simulink model "busCreators01curr"  (R2025b)
settings: Solver=VariableStepAuto  StartTime=0.0  StopTime=10.0  RelTol=1e-3
undefined symbols (not defined in the file or in its folder): Ts
settings Model: Creator=gdudgeon  LastModifiedBy=gdudgeon
settings RTWCC: GPUComputeCapability=3.5

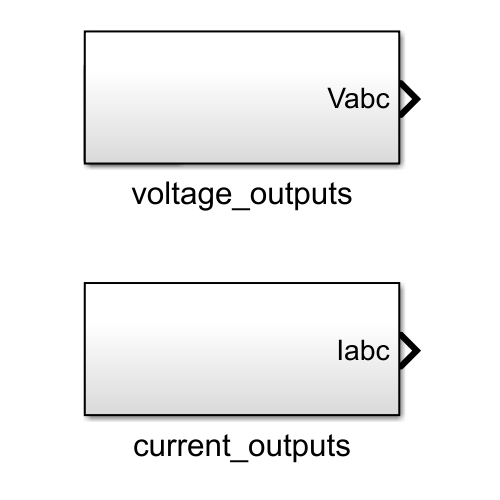
[thumbnail: Simulink's stored preview of the top-level diagram]
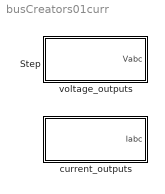
== system busCreators01curr ==
  Step : Step  SampleTime=0
  current_outputs : Subsystem
  voltage_outputs : Subsystem

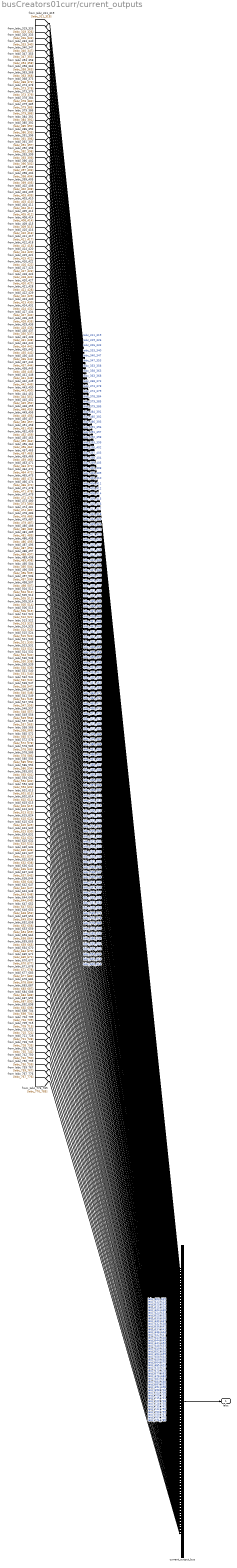
== system busCreators01curr/current_outputs ==
  current_output_bus : BusCreator  Inputs=169
  Iabc : Outport  SampleTime=Ts  VectorParamsAs1DForOutWhenUnconnected=off
  wires:
  [Iabc_776_785] -> current_output_bus/169  "Iabc_776_785"
  [Iabc_767_776] -> current_output_bus/168  "Iabc_767_776"
  [Iabc_759_767] -> current_output_bus/167  "Iabc_759_767"
  [Iabc_750_759] -> current_output_bus/166  "Iabc_750_759"
  [Iabc_742_750] -> current_output_bus/165  "Iabc_742_750"
  [Iabc_735_742] -> current_output_bus/164  "Iabc_735_742"
  [Iabc_728_735] -> current_output_bus/163  "Iabc_728_735"
  [Iabc_721_728] -> current_output_bus/162  "Iabc_721_728"
  [Iabc_715_721] -> current_output_bus/161  "Iabc_715_721"
  [Iabc_709_715] -> current_output_bus/160  "Iabc_709_715"
  [Iabc_704_709] -> current_output_bus/159  "Iabc_704_709"
  [Iabc_698_704] -> current_output_bus/158  "Iabc_698_704"
  [Iabc_692_698] -> current_output_bus/157  "Iabc_692_698"
  [Iabc_687_692] -> current_output_bus/156  "Iabc_687_692"
  [Iabc_684_688] -> current_output_bus/155  "Iabc_684_688"
  [Iabc_683_687] -> current_output_bus/154  "Iabc_683_687"
  [Iabc_678_684] -> current_output_bus/153  "Iabc_678_684"
  [Iabc_677_683] -> current_output_bus/152  "Iabc_677_683"
  [Iabc_671_678] -> current_output_bus/151  "Iabc_671_678"
  [Iabc_670_677] -> current_output_bus/150  "Iabc_670_677"
  [Iabc_665_671] -> current_output_bus/149  "Iabc_665_671"
  [Iabc_664_670] -> current_output_bus/148  "Iabc_664_670"
  [Iabc_659_665] -> current_output_bus/147  "Iabc_659_665"
  [Iabc_658_664] -> current_output_bus/146  "Iabc_658_664"
  [Iabc_653_659] -> current_output_bus/145  "Iabc_653_659"
  [Iabc_652_658] -> current_output_bus/144  "Iabc_652_658"
  [Iabc_649_654] -> current_output_bus/143  "Iabc_649_654"
  [Iabc_648_653] -> current_output_bus/142  "Iabc_648_653"
  [Iabc_647_652] -> current_output_bus/141  "Iabc_647_652"
  [Iabc_644_649] -> current_output_bus/140  "Iabc_644_649"
  [Iabc_643_648] -> current_output_bus/139  "Iabc_643_648"
  [Iabc_642_647] -> current_output_bus/138  "Iabc_642_647"
  [Iabc_638_644] -> current_output_bus/137  "Iabc_638_644"
  [Iabc_637_643] -> current_output_bus/136  "Iabc_637_643"
  [Iabc_636_642] -> current_output_bus/135  "Iabc_636_642"
  [Iabc_632_638] -> current_output_bus/134  "Iabc_632_638"
  [Iabc_631_637] -> current_output_bus/133  "Iabc_631_637"
  [Iabc_630_636] -> current_output_bus/132  "Iabc_630_636"
  [Iabc_625_632] -> current_output_bus/131  "Iabc_625_632"
  [Iabc_624_631] -> current_output_bus/130  "Iabc_624_631"
  [Iabc_623_630] -> current_output_bus/129  "Iabc_623_630"
  [Iabc_615_625] -> current_output_bus/128  "Iabc_615_625"
  [Iabc_615_624] -> current_output_bus/127  "Iabc_615_624"
  [Iabc_613_623] -> current_output_bus/126  "Iabc_613_623"
  [Iabc_603_615] -> current_output_bus/125  "Iabc_603_615"
  [Iabc_602_614] -> current_output_bus/124  "Iabc_602_614"
  [Iabc_601_613] -> current_output_bus/123  "Iabc_601_613"
  [Iabc_594_603] -> current_output_bus/122  "Iabc_594_603"
  [Iabc_594_602] -> current_output_bus/121  "Iabc_594_602"
  [Iabc_593_601] -> current_output_bus/120  "Iabc_593_601"
  [Iabc_586_594] -> current_output_bus/119  "Iabc_586_594"
  [Iabc_585_593] -> current_output_bus/118  "Iabc_585_593"
  [Iabc_578_586] -> current_output_bus/117  "Iabc_578_586"
  [Iabc_578_585] -> current_output_bus/116  "Iabc_578_585"
  [Iabc_572_578] -> current_output_bus/115  "Iabc_572_578"
  [Iabc_565_572] -> current_output_bus/114  "Iabc_565_572"
  [Iabc_558_566] -> current_output_bus/113  "Iabc_558_566"
  [Iabc_557_565] -> current_output_bus/112  "Iabc_557_565"
  [Iabc_549_558] -> current_output_bus/111  "Iabc_549_558"
  [Iabc_548_557] -> current_output_bus/110  "Iabc_548_557"
  [Iabc_547_556] -> current_output_bus/109  "Iabc_547_556"
  [Iabc_541_549] -> current_output_bus/108  "Iabc_541_549"
  [Iabc_540_548] -> current_output_bus/107  "Iabc_540_548"
  [Iabc_538_547] -> current_output_bus/106  "Iabc_538_547"
  [Iabc_532_541] -> current_output_bus/105  "Iabc_532_541"
  [Iabc_531_540] -> current_output_bus/104  "Iabc_531_540"
  [Iabc_530_539] -> current_output_bus/103  "Iabc_530_539"
  [Iabc_530_538] -> current_output_bus/102  "Iabc_530_538"
  [Iabc_524_532] -> current_output_bus/101  "Iabc_524_532"
  [Iabc_523_531] -> current_output_bus/100  "Iabc_523_531"
  [Iabc_521_530] -> current_output_bus/99  "Iabc_521_530"
  [Iabc_515_524] -> current_output_bus/98  "Iabc_515_524"
  [Iabc_514_523] -> current_output_bus/97  "Iabc_514_523"
  [Iabc_513_522] -> current_output_bus/96  "Iabc_513_522"
  [Iabc_512_521] -> current_output_bus/95  "Iabc_512_521"
  [Iabc_506_515] -> current_output_bus/94  "Iabc_506_515"
  [Iabc_505_514] -> current_output_bus/93  "Iabc_505_514"
  [Iabc_505_513] -> current_output_bus/92  "Iabc_505_513"
  [Iabc_504_512] -> current_output_bus/91  "Iabc_504_512"
  [Iabc_498_507] -> current_output_bus/90  "Iabc_498_507"
  [Iabc_497_506] -> current_output_bus/89  "Iabc_497_506"
  [Iabc_496_505] -> current_output_bus/88  "Iabc_496_505"
  [Iabc_495_504] -> current_output_bus/87  "Iabc_495_504"
  [Iabc_489_498] -> current_output_bus/86  "Iabc_489_498"
  [Iabc_488_497] -> current_output_bus/85  "Iabc_488_497"
  [Iabc_487_496] -> current_output_bus/84  "Iabc_487_496"
  [Iabc_486_495] -> current_output_bus/83  "Iabc_486_495"
  [Iabc_481_489] -> current_output_bus/82  "Iabc_481_489"
  [Iabc_480_488] -> current_output_bus/81  "Iabc_480_488"
  [Iabc_479_487] -> current_output_bus/80  "Iabc_479_487"
  [Iabc_478_486] -> current_output_bus/79  "Iabc_478_486"
  [Iabc_474_481] -> current_output_bus/78  "Iabc_474_481"
  [Iabc_473_480] -> current_output_bus/77  "Iabc_473_480"
  [Iabc_472_479] -> current_output_bus/76  "Iabc_472_479"
  [Iabc_471_478] -> current_output_bus/75  "Iabc_471_478"
  [Iabc_466_474] -> current_output_bus/74  "Iabc_466_474"
  [Iabc_465_473] -> current_output_bus/73  "Iabc_465_473"
  [Iabc_464_472] -> current_output_bus/72  "Iabc_464_472"
  [Iabc_463_471] -> current_output_bus/71  "Iabc_463_471"
  [Iabc_459_466] -> current_output_bus/70  "Iabc_459_466"
  [Iabc_457_465] -> current_output_bus/69  "Iabc_457_465"
  [Iabc_456_464] -> current_output_bus/68  "Iabc_456_464"
  [Iabc_455_463] -> current_output_bus/67  "Iabc_455_463"
  [Iabc_452_459] -> current_output_bus/66  "Iabc_452_459"
  [Iabc_451_458] -> current_output_bus/65  "Iabc_451_458"
  [Iabc_450_457] -> current_output_bus/64  "Iabc_450_457"
  [Iabc_449_456] -> current_output_bus/63  "Iabc_449_456"
  [Iabc_448_455] -> current_output_bus/62  "Iabc_448_455"
  [Iabc_445_452] -> current_output_bus/61  "Iabc_445_452"
  [Iabc_444_451] -> current_output_bus/60  "Iabc_444_451"
  [Iabc_443_450] -> current_output_bus/59  "Iabc_443_450"
  [Iabc_442_449] -> current_output_bus/58  "Iabc_442_449"
  [Iabc_441_448] -> current_output_bus/57  "Iabc_441_448"
  [Iabc_438_445] -> current_output_bus/56  "Iabc_438_445"
  [Iabc_437_444] -> current_output_bus/55  "Iabc_437_444"
  [Iabc_436_443] -> current_output_bus/54  "Iabc_436_443"
  [Iabc_435_442] -> current_output_bus/53  "Iabc_435_442"
  [Iabc_434_441] -> current_output_bus/52  "Iabc_434_441"
  [Iabc_431_438] -> current_output_bus/51  "Iabc_431_438"
  [Iabc_430_437] -> current_output_bus/50  "Iabc_430_437"
  [Iabc_429_436] -> current_output_bus/49  "Iabc_429_436"
  [Iabc_428_435] -> current_output_bus/48  "Iabc_428_435"
  [Iabc_427_434] -> current_output_bus/47  "Iabc_427_434"
  [Iabc_424_431] -> current_output_bus/46  "Iabc_424_431"
  [Iabc_423_430] -> current_output_bus/45  "Iabc_423_430"
  [Iabc_422_429] -> current_output_bus/44  "Iabc_422_429"
  [Iabc_421_428] -> current_output_bus/43  "Iabc_421_428"
  [Iabc_420_427] -> current_output_bus/42  "Iabc_420_427"
  [Iabc_418_424] -> current_output_bus/41  "Iabc_418_424"
  [Iabc_417_423] -> current_output_bus/40  "Iabc_417_423"
  [Iabc_416_422] -> current_output_bus/39  "Iabc_416_422"
  [Iabc_415_421] -> current_output_bus/38  "Iabc_415_421"
  [Iabc_414_420] -> current_output_bus/37  "Iabc_414_420"
  [Iabc_412_418] -> current_output_bus/36  "Iabc_412_418"
  [Iabc_411_417] -> current_output_bus/35  "Iabc_411_417"
  [Iabc_410_416] -> current_output_bus/34  "Iabc_410_416"
  [Iabc_409_415] -> current_output_bus/33  "Iabc_409_415"
  [Iabc_408_414] -> current_output_bus/32  "Iabc_408_414"
  [Iabc_405_412] -> current_output_bus/31  "Iabc_405_412"
  [Iabc_404_411] -> current_output_bus/30  "Iabc_404_411"
  [Iabc_403_410] -> current_output_bus/29  "Iabc_403_410"
  [Iabc_403_409] -> current_output_bus/28  "Iabc_403_409"
  [Iabc_402_408] -> current_output_bus/27  "Iabc_402_408"
  [Iabc_399_405] -> current_output_bus/26  "Iabc_399_405"
  [Iabc_398_404] -> current_output_bus/25  "Iabc_398_404"
  [Iabc_397_403] -> current_output_bus/24  "Iabc_397_403"
  [Iabc_396_402] -> current_output_bus/23  "Iabc_396_402"
  [Iabc_393_399] -> current_output_bus/22  "Iabc_393_399"
  [Iabc_392_398] -> current_output_bus/21  "Iabc_392_398"
  [Iabc_391_397] -> current_output_bus/20  "Iabc_391_397"
  [Iabc_391_396] -> current_output_bus/19  "Iabc_391_396"
  [Iabc_386_393] -> current_output_bus/18  "Iabc_386_393"
  [Iabc_385_392] -> current_output_bus/17  "Iabc_385_392"
  [Iabc_384_391] -> current_output_bus/16  "Iabc_384_391"
  [Iabc_379_386] -> current_output_bus/15  "Iabc_379_386"
  [Iabc_379_385] -> current_output_bus/14  "Iabc_379_385"
  [Iabc_378_384] -> current_output_bus/13  "Iabc_378_384"
  [Iabc_373_379] -> current_output_bus/12  "Iabc_373_379"
  [Iabc_373_378] -> current_output_bus/11  "Iabc_373_378"
  [Iabc_368_373] -> current_output_bus/10  "Iabc_368_373"
  [Iabc_363_368] -> current_output_bus/9  "Iabc_363_368"
  [Iabc_358_363] -> current_output_bus/8  "Iabc_358_363"
  [Iabc_353_358] -> current_output_bus/7  "Iabc_353_358"
  [Iabc_347_353] -> current_output_bus/6  "Iabc_347_353"
  [Iabc_340_347] -> current_output_bus/5  "Iabc_340_347"
  [Iabc_333_340] -> current_output_bus/4  "Iabc_333_340"
  [Iabc_326_333] -> current_output_bus/3  "Iabc_326_333"
  [Iabc_319_326] -> current_output_bus/2  "Iabc_319_326"
  [Iabc_311_319] -> current_output_bus/1  "Iabc_311_319"
  current_output_bus/1 -> Iabc/1

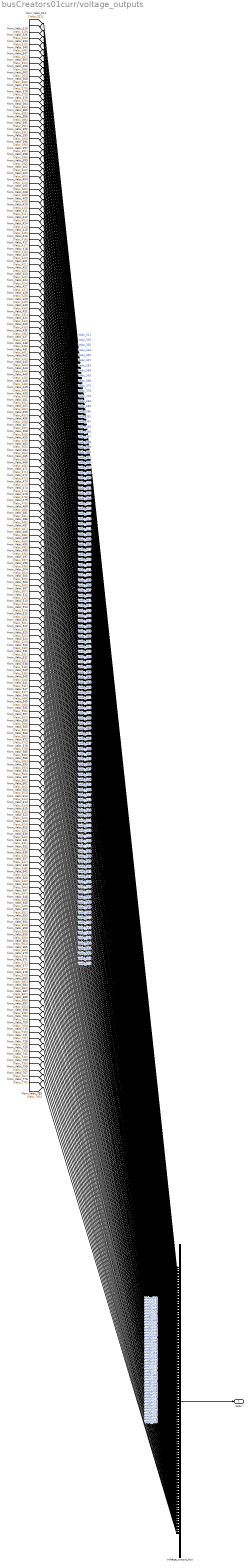
== system busCreators01curr/voltage_outputs ==
  voltage_output_bus : BusCreator  Inputs=170
  Vabc : Outport  SampleTime=Ts  VectorParamsAs1DForOutWhenUnconnected=off
  wires:
  [Vabc_785] -> voltage_output_bus/170  "Vabc_785"
  [Vabc_776] -> voltage_output_bus/169  "Vabc_776"
  [Vabc_767] -> voltage_output_bus/168  "Vabc_767"
  [Vabc_759] -> voltage_output_bus/167  "Vabc_759"
  [Vabc_750] -> voltage_output_bus/166  "Vabc_750"
  [Vabc_742] -> voltage_output_bus/165  "Vabc_742"
  [Vabc_735] -> voltage_output_bus/164  "Vabc_735"
  [Vabc_728] -> voltage_output_bus/163  "Vabc_728"
  [Vabc_721] -> voltage_output_bus/162  "Vabc_721"
  [Vabc_715] -> voltage_output_bus/161  "Vabc_715"
  [Vabc_709] -> voltage_output_bus/160  "Vabc_709"
  [Vabc_704] -> voltage_output_bus/159  "Vabc_704"
  [Vabc_698] -> voltage_output_bus/158  "Vabc_698"
  [Vabc_692] -> voltage_output_bus/157  "Vabc_692"
  [Vabc_688] -> voltage_output_bus/156  "Vabc_688"
  [Vabc_687] -> voltage_output_bus/155  "Vabc_687"
  [Vabc_684] -> voltage_output_bus/154  "Vabc_684"
  [Vabc_683] -> voltage_output_bus/153  "Vabc_683"
  [Vabc_678] -> voltage_output_bus/152  "Vabc_678"
  [Vabc_677] -> voltage_output_bus/151  "Vabc_677"
  [Vabc_671] -> voltage_output_bus/150  "Vabc_671"
  [Vabc_670] -> voltage_output_bus/149  "Vabc_670"
  [Vabc_665] -> voltage_output_bus/148  "Vabc_665"
  [Vabc_664] -> voltage_output_bus/147  "Vabc_664"
  [Vabc_659] -> voltage_output_bus/146  "Vabc_659"
  [Vabc_658] -> voltage_output_bus/145  "Vabc_658"
  [Vabc_654] -> voltage_output_bus/144  "Vabc_654"
  [Vabc_653] -> voltage_output_bus/143  "Vabc_653"
  [Vabc_652] -> voltage_output_bus/142  "Vabc_652"
  [Vabc_649] -> voltage_output_bus/141  "Vabc_649"
  [Vabc_648] -> voltage_output_bus/140  "Vabc_648"
  [Vabc_647] -> voltage_output_bus/139  "Vabc_647"
  [Vabc_644] -> voltage_output_bus/138  "Vabc_644"
  [Vabc_643] -> voltage_output_bus/137  "Vabc_643"
  [Vabc_642] -> voltage_output_bus/136  "Vabc_642"
  [Vabc_638] -> voltage_output_bus/135  "Vabc_638"
  [Vabc_637] -> voltage_output_bus/134  "Vabc_637"
  [Vabc_636] -> voltage_output_bus/133  "Vabc_636"
  [Vabc_632] -> voltage_output_bus/132  "Vabc_632"
  [Vabc_631] -> voltage_output_bus/131  "Vabc_631"
  [Vabc_630] -> voltage_output_bus/130  "Vabc_630"
  [Vabc_625] -> voltage_output_bus/129  "Vabc_625"
  [Vabc_624] -> voltage_output_bus/128  "Vabc_624"
  [Vabc_623] -> voltage_output_bus/127  "Vabc_623"
  [Vabc_615] -> voltage_output_bus/126  "Vabc_615"
  [Vabc_614] -> voltage_output_bus/125  "Vabc_614"
  [Vabc_613] -> voltage_output_bus/124  "Vabc_613"
  [Vabc_603] -> voltage_output_bus/123  "Vabc_603"
  [Vabc_602] -> voltage_output_bus/122  "Vabc_602"
  [Vabc_601] -> voltage_output_bus/121  "Vabc_601"
  [Vabc_594] -> voltage_output_bus/120  "Vabc_594"
  [Vabc_593] -> voltage_output_bus/119  "Vabc_593"
  [Vabc_586] -> voltage_output_bus/118  "Vabc_586"
  [Vabc_585] -> voltage_output_bus/117  "Vabc_585"
  [Vabc_578] -> voltage_output_bus/116  "Vabc_578"
  [Vabc_572] -> voltage_output_bus/115  "Vabc_572"
  [Vabc_566] -> voltage_output_bus/114  "Vabc_566"
  [Vabc_565] -> voltage_output_bus/113  "Vabc_565"
  [Vabc_558] -> voltage_output_bus/112  "Vabc_558"
  [Vabc_557] -> voltage_output_bus/111  "Vabc_557"
  [Vabc_556] -> voltage_output_bus/110  "Vabc_556"
  [Vabc_549] -> voltage_output_bus/109  "Vabc_549"
  [Vabc_548] -> voltage_output_bus/108  "Vabc_548"
  [Vabc_547] -> voltage_output_bus/107  "Vabc_547"
  [Vabc_541] -> voltage_output_bus/106  "Vabc_541"
  [Vabc_540] -> voltage_output_bus/105  "Vabc_540"
  [Vabc_539] -> voltage_output_bus/104  "Vabc_539"
  [Vabc_538] -> voltage_output_bus/103  "Vabc_538"
  [Vabc_532] -> voltage_output_bus/102  "Vabc_532"
  [Vabc_531] -> voltage_output_bus/101  "Vabc_531"
  [Vabc_530] -> voltage_output_bus/100  "Vabc_530"
  [Vabc_524] -> voltage_output_bus/99  "Vabc_524"
  [Vabc_523] -> voltage_output_bus/98  "Vabc_523"
  [Vabc_522] -> voltage_output_bus/97  "Vabc_522"
  [Vabc_521] -> voltage_output_bus/96  "Vabc_521"
  [Vabc_515] -> voltage_output_bus/95  "Vabc_515"
  [Vabc_514] -> voltage_output_bus/94  "Vabc_514"
  [Vabc_513] -> voltage_output_bus/93  "Vabc_513"
  [Vabc_512] -> voltage_output_bus/92  "Vabc_512"
  [Vabc_507] -> voltage_output_bus/91  "Vabc_507"
  [Vabc_506] -> voltage_output_bus/90  "Vabc_506"
  [Vabc_505] -> voltage_output_bus/89  "Vabc_505"
  [Vabc_504] -> voltage_output_bus/88  "Vabc_504"
  [Vabc_498] -> voltage_output_bus/87  "Vabc_498"
  [Vabc_497] -> voltage_output_bus/86  "Vabc_497"
  [Vabc_496] -> voltage_output_bus/85  "Vabc_496"
  [Vabc_495] -> voltage_output_bus/84  "Vabc_495"
  [Vabc_489] -> voltage_output_bus/83  "Vabc_489"
  [Vabc_488] -> voltage_output_bus/82  "Vabc_488"
  [Vabc_487] -> voltage_output_bus/81  "Vabc_487"
  [Vabc_486] -> voltage_output_bus/80  "Vabc_486"
  [Vabc_481] -> voltage_output_bus/79  "Vabc_481"
  [Vabc_480] -> voltage_output_bus/78  "Vabc_480"
  [Vabc_479] -> voltage_output_bus/77  "Vabc_479"
  [Vabc_478] -> voltage_output_bus/76  "Vabc_478"
  [Vabc_474] -> voltage_output_bus/75  "Vabc_474"
  [Vabc_473] -> voltage_output_bus/74  "Vabc_473"
  [Vabc_472] -> voltage_output_bus/73  "Vabc_472"
  [Vabc_471] -> voltage_output_bus/72  "Vabc_471"
  [Vabc_466] -> voltage_output_bus/71  "Vabc_466"
  [Vabc_465] -> voltage_output_bus/70  "Vabc_465"
  [Vabc_464] -> voltage_output_bus/69  "Vabc_464"
  [Vabc_463] -> voltage_output_bus/68  "Vabc_463"
  [Vabc_459] -> voltage_output_bus/67  "Vabc_459"
  [Vabc_458] -> voltage_output_bus/66  "Vabc_458"
  [Vabc_457] -> voltage_output_bus/65  "Vabc_457"
  [Vabc_456] -> voltage_output_bus/64  "Vabc_456"
  [Vabc_455] -> voltage_output_bus/63  "Vabc_455"
  [Vabc_452] -> voltage_output_bus/62  "Vabc_452"
  [Vabc_451] -> voltage_output_bus/61  "Vabc_451"
  [Vabc_450] -> voltage_output_bus/60  "Vabc_450"
  [Vabc_449] -> voltage_output_bus/59  "Vabc_449"
  [Vabc_448] -> voltage_output_bus/58  "Vabc_448"
  [Vabc_445] -> voltage_output_bus/57  "Vabc_445"
  [Vabc_444] -> voltage_output_bus/56  "Vabc_444"
  [Vabc_443] -> voltage_output_bus/55  "Vabc_443"
  [Vabc_442] -> voltage_output_bus/54  "Vabc_442"
  [Vabc_441] -> voltage_output_bus/53  "Vabc_441"
  [Vabc_438] -> voltage_output_bus/52  "Vabc_438"
  [Vabc_437] -> voltage_output_bus/51  "Vabc_437"
  [Vabc_436] -> voltage_output_bus/50  "Vabc_436"
  [Vabc_435] -> voltage_output_bus/49  "Vabc_435"
  [Vabc_434] -> voltage_output_bus/48  "Vabc_434"
  [Vabc_431] -> voltage_output_bus/47  "Vabc_431"
  [Vabc_430] -> voltage_output_bus/46  "Vabc_430"
  [Vabc_429] -> voltage_output_bus/45  "Vabc_429"
  [Vabc_428] -> voltage_output_bus/44  "Vabc_428"
  [Vabc_427] -> voltage_output_bus/43  "Vabc_427"
  [Vabc_424] -> voltage_output_bus/42  "Vabc_424"
  [Vabc_423] -> voltage_output_bus/41  "Vabc_423"
  [Vabc_422] -> voltage_output_bus/40  "Vabc_422"
  [Vabc_421] -> voltage_output_bus/39  "Vabc_421"
  [Vabc_420] -> voltage_output_bus/38  "Vabc_420"
  [Vabc_418] -> voltage_output_bus/37  "Vabc_418"
  [Vabc_417] -> voltage_output_bus/36  "Vabc_417"
  [Vabc_416] -> voltage_output_bus/35  "Vabc_416"
  [Vabc_415] -> voltage_output_bus/34  "Vabc_415"
  [Vabc_414] -> voltage_output_bus/33  "Vabc_414"
  [Vabc_412] -> voltage_output_bus/32  "Vabc_412"
  [Vabc_411] -> voltage_output_bus/31  "Vabc_411"
  [Vabc_410] -> voltage_output_bus/30  "Vabc_410"
  [Vabc_409] -> voltage_output_bus/29  "Vabc_409"
  [Vabc_408] -> voltage_output_bus/28  "Vabc_408"
  [Vabc_405] -> voltage_output_bus/27  "Vabc_405"
  [Vabc_404] -> voltage_output_bus/26  "Vabc_404"
  [Vabc_403] -> voltage_output_bus/25  "Vabc_403"
  [Vabc_402] -> voltage_output_bus/24  "Vabc_402"
  [Vabc_399] -> voltage_output_bus/23  "Vabc_399"
  [Vabc_398] -> voltage_output_bus/22  "Vabc_398"
  [Vabc_397] -> voltage_output_bus/21  "Vabc_397"
  [Vabc_396] -> voltage_output_bus/20  "Vabc_396"
  [Vabc_393] -> voltage_output_bus/19  "Vabc_393"
  [Vabc_392] -> voltage_output_bus/18  "Vabc_392"
  [Vabc_391] -> voltage_output_bus/17  "Vabc_391"
  [Vabc_386] -> voltage_output_bus/16  "Vabc_386"
  [Vabc_385] -> voltage_output_bus/15  "Vabc_385"
  [Vabc_384] -> voltage_output_bus/14  "Vabc_384"
  [Vabc_379] -> voltage_output_bus/13  "Vabc_379"
  [Vabc_378] -> voltage_output_bus/12  "Vabc_378"
  [Vabc_373] -> voltage_output_bus/11  "Vabc_373"
  [Vabc_368] -> voltage_output_bus/10  "Vabc_368"
  [Vabc_363] -> voltage_output_bus/9  "Vabc_363"
  [Vabc_358] -> voltage_output_bus/8  "Vabc_358"
  [Vabc_353] -> voltage_output_bus/7  "Vabc_353"
  [Vabc_347] -> voltage_output_bus/6  "Vabc_347"
  [Vabc_340] -> voltage_output_bus/5  "Vabc_340"
  [Vabc_333] -> voltage_output_bus/4  "Vabc_333"
  [Vabc_326] -> voltage_output_bus/3  "Vabc_326"
  [Vabc_319] -> voltage_output_bus/2  "Vabc_319"
  [Vabc_311] -> voltage_output_bus/1  "Vabc_311"
  voltage_output_bus/1 -> Vabc/1
